simulink model "model_demo"  (R2023b)
settings: Solver=VariableStepAuto  StartTime=0.0  StopTime=10.0  RelTol=1e-3
undefined symbols (not defined in the file): DiscIntNeverNeededParam, magnitude, Newton, Raphson
libraries: simulink x61, slpidlib x19
(part 1 of 3)
settings Model: Creator=OSCAR4  LastModifiedBy=OSCAR4

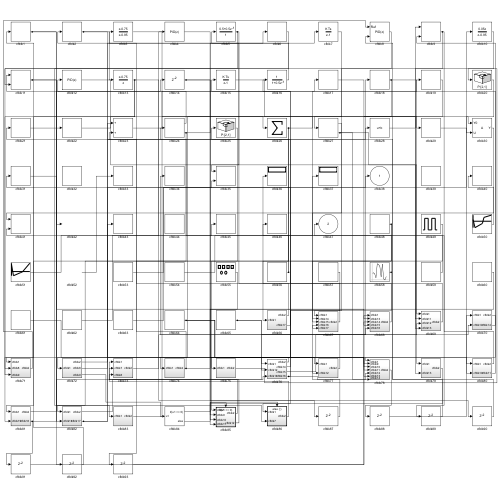
[thumbnail: Simulink's stored preview of the top-level diagram]
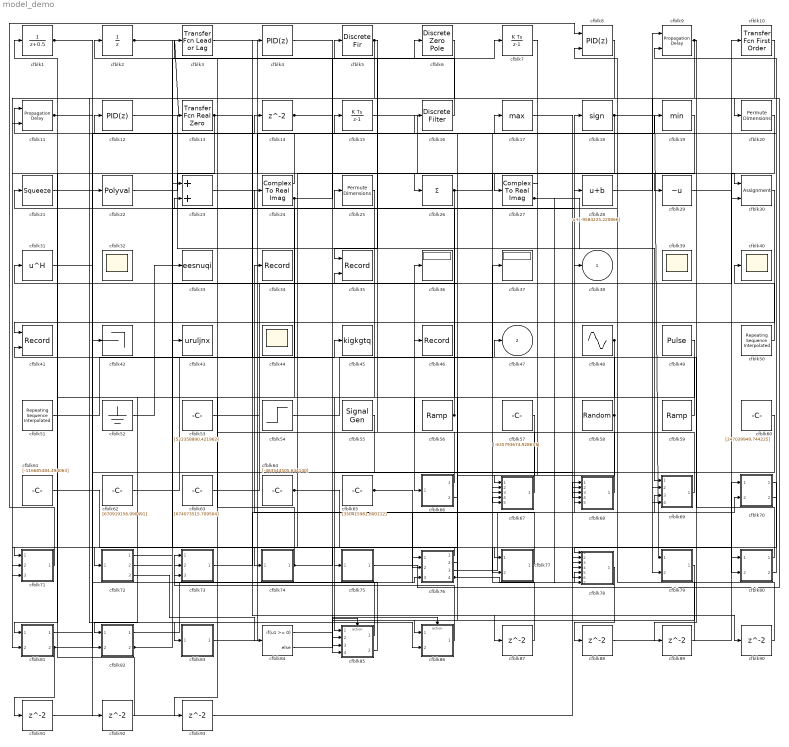
== system model_demo ==
  cfblk1 : DiscreteTransferFcn  SampleTime=1
  cfblk10 : simulink/Discrete/Transfer Fcn First Order  PoleZ=0.95  ICPrevOutput=0.0  DoSatur=off
  cfblk11 : PropagationDelay  SampleTime=1
  cfblk12 : slpidlib/PID Controller  Controller=PID  Form=Parallel  TimeDomain=Discrete-time  UseExternalTs=off  SampleTime=1  IntegratorMethod=Forward Euler  FilterMethod=Forward Euler  ControllerParametersSource=internal  P=1  I=1  UseKiTs=off  D=0  N=100  UseFilter=on  TunerSelectOption=Transfer Function Based (PID Tuner App)  InitialConditionSource=internal  InitialConditionForIntegrator=0  InitialConditionForFilter=0  DifferentiatorICPrevScaledInput=0  ExternalReset=none  TrackingMode=off  Kt=1  LimitOutput=off  SatLimitsSource=internal  UpperSaturationLimit=inf  LowerSaturationLimit=-inf  LinearizeAsGain=off  AntiWindupMode=none  Kb=1  LimitIntegrator=off  UpperIntegratorSaturationLimit=inf  LowerIntegratorSaturationLimit=-inf  POutMin=[]  POutMax=[]  IOutMin=[]  IOutMax=[]  DOutMin=[]  DOutMax=[]  NOutMin=[]  NOutMax=[]  SumOutMin=[]  SumOutMax=[]  SaturationOutMin=[]  SaturationOutMax=[]  PParamMin=[]  PParamMax=[]  IParamMin=[]  IParamMax=[]  DParamMin=[]  DParamMax=[]  NParamMin=[]  NParamMax=[]  KbParamMin=[]  KbParamMax=[]  KtParamMin=[]  KtParamMax=[]  KbOutMin=[]  KbOutMax=[]  KtOutMin=[]  KtOutMax=[]  IntegratorOutMin=[]  IntegratorOutMax=[]  FilterOutMin=[]  FilterOutMax=[]  SumI1OutMin=[]  SumI1OutMax=[]  SumI2OutMin=[]  SumI2OutMax=[]  SumI3OutMin=[]  SumI3OutMax=[]  SumI4OutMin=[]  SumI4OutMax=[]  SumDOutMin=[]  SumDOutMax=[]  DifferentiatorOutMin=[]  DifferentiatorOutMax=[]  FilterDiffOutCoefMin=[]  FilterDiffOutCoefMax=[]  ReciprocalOutMin=[]  ReciprocalOutMax=[]  SumDenOutMin=[]  SumDenOutMax=[]  SumNumOutMin=[]  SumNumOutMax=[]  DivideOutMin=[]  DivideOutMax=[]  UdiffTsProdOutMin=[]  UdiffTsProdOutMax=[]  NTsProdOutMin=[]  NTsProdOutMax=[]  UintegralTsProdOutMin=[]  UintegralTsProdOutMax=[]  UngainTsProdOutMin=[]  UngainTsProdOutMax=[]  ClampingZeroOutDataTypeStr=Inherit: Inherit via back propagation  ClampingZeroOutMin=[]  ClampingZeroOutMax=[]  FilterDenConstantOutDataTypeStr=Inherit: Inherit via back propagation  FilterDenConstantOutMin=[]  FilterDenConstantOutMax=[]  PCopyOutDataTypeStr=Inherit: Inherit via back propagation  PCopyOutMin=[]  PCopyOutMax=[]  NCopyOutDataTypeStr=Inherit: Inherit via back propagation  NCopyOutMin=[]  NCopyOutMax=[]  IntegratorContinuousStateAttributes=''  IntegratorStateMustResolveToSignalObject=off  IntegratorRTWStateStorageClass=Auto  FilterContinuousStateAttributes=''  FilterStateMustResolveToSignalObject=off  FilterRTWStateStorageClass=Auto  ParallelPVariant=InternalParameters  IdealPVariant=Disabled  IVariant=InternalParameters  DVariant=InternalParameters  IntegratorVariant=Discrete  SatVariant=Disabled  AWVariant=Passthrough  PCopyVariant=Disabled  TRVariant=Disabled  FdbkBlocksVariant=Forward  IdealPFdbkVariant=Disabled  SatFdbkVariant=Disabled  DerivativeFilterVariant=ForwardEulerFilter  NVariant=InternalParameters  NCopyVariant=Disabled  FilterICVariant=InternalICsFilter  IntegratorICVariant=InternalICs  ExternalResetVariant=Disabled  TRSumVariant=Passthrough  SumFdbkVariant=Disabled  SumVariant=Sum_PID  TsampFilterVariant=InternalTs  TsampNgainVariant=Passthrough  TsampIntegralVariant=Disabled_SignalSpec  ExternalSaturationOutDataTypeStr=Inherit: Same as second input
      settings: LibrarySourceBlock=simulink/Discrete/Discrete PID Controller
  cfblk13 : simulink/Discrete/Transfer Fcn Real Zero  ZeroZ=0.75  ICPrevInput=0.0  DoSatur=off
  cfblk{14,87..93} (8 alike) : Delay  SampleTime=1
  cfblk15 : DiscreteIntegrator  ICPrevOutput=DiscIntNeverNeededParam  ICPrevScaledInput=DiscIntNeverNeededParam
  cfblk16 : DiscreteFilter  SampleTime=1
  cfblk17 : MinMax  Function=max
  cfblk18 : Signum
  cfblk19 : MinMax
  cfblk2 : UnitDelay  HasFrameUpgradeWarning=on
  cfblk20 : PermuteDimensions
  cfblk21 : Squeeze
  cfblk22 : Polyval  Coefs=[ +2.081618890e-019, -1.441693666e-014, +4.719686976e-010, -8.536869453e-006, +1.621573104e-001, -8.087801117e+001 ]
  cfblk23 : Sum
  cfblk24 : ComplexToRealImag
  cfblk25 : PermuteDimensions
  cfblk26 : Sum  Inputs=+
  cfblk27 : ComplexToRealImag
  cfblk28 : Bias  Bias=[-9584225.220866]  SaturateOnIntegerOverflow=off
  cfblk29 : UnaryMinus
  cfblk3 : simulink/Discrete/Transfer Fcn Lead or Lag  PoleZ=0.95  ZeroZ=0.75  ICPrevOutput=0.0  ICPrevInput=0.0  DoSatur=off
  cfblk30 : Assignment  DiagnosticForDimensions=Warning  IndexOptions=Index vector (dialog)  Indices=1  OutputSizes=1
  cfblk31 : Math  Operator=hermitian
  cfblk{32,39..40,44} (4 alike) : Scope
      cfblk32 settings: Floating=on
      cfblk39 settings: Floating=on
      cfblk44 settings: Floating=on
  cfblk33 : ToWorkspace  VariableName=eesnuqi  SaveFormat=Timeseries  SampleTime=-1
  cfblk34 : Record  FileSettingsInternal="{\"entries\":[{\"content\":{\"excelSettings\":{\"content\":{},\"type\":\"Streamout.ExcelSettings\"}},\"type\":\"Streamout.FileSettingStorage\",\"uuid\":\"\"}],\"packageUris\":[\"http:\\/\\/schema.mathworks.com\\/mf0\\/streamout_blocks\\/R2020a\"],\"version\":\"1.0\"}"  SignalsInternal="{\"entries\":[{\"content\":{},\"type\":\"RecordBlkView.InputSignals\",\"uuid\":\"\"}],\"packageUris\":[\"http:\\/\\/schema.mathworks.com\\/mf0\\/streamout_blocks\\/R2020a\"],\"version\":\"1.0\"}"  VisualizationBindings="{\"sparklinesplugin\":{\"info\":[{\"bindingParametersList\":[],\"subplotID\":1}]}}"
  cfblk35 : Record  FileSettingsInternal="{\"entries\":[{\"content\":{\"excelSettings\":{\"content\":{},\"type\":\"Streamout.ExcelSettings\"}},\"type\":\"Streamout.FileSettingStorage\",\"uuid\":\"\"}],\"packageUris\":[\"http:\\/\\/schema.mathworks.com\\/mf0\\/streamout_blocks\\/R2020a\"],\"version\":\"1.0\"}"  Layout=[1 1]  SignalsInternal="{\"entries\":[{\"content\":{\"signals\":[{\"content\":{\"blockPath\":[],\"dimensions\":[1],\"domain\":\"\",\"lineColor\":\"#a2142f\",\"plots\":[1],\"port\":1,\"signalID\":7067,\"signalName\":\"XY Graph:1\"},\"type\":\"RecordBlkView.Signal\",\"uuid\":\"\"},{\"content\":{\"blockPath\":[],\"dimensions\":[1],\"domain\":\"\",\"lineColor\":\"#139fff\",\"plots\":[1],\"port\":2,\"signalID\":7070,\"signalName\":\"XY Graph:2\"},\"type\":\"RecordBlkView.Signal\",\"uuid\":\"\"}]},\"type\":\"RecordBlkView.InputSignals\",\"uuid\":\"\"}],\"packageUris\":[\"http:\\/\\/schema.mathworks.com\\/mf0\\/streamout_blocks\\/R2020a\"],\"version\":\"1.0\"}"  VisualizationBindings="{\"xyplotplugin\":{\"info\":[{\"series\":[{\"bindingParametersList\":[{\"parameter\":\"X-Axis\",\"signalID\":7067,\"signalName\":\"XY Graph:1\"},{\"parameter\":\"Y-Axis\",\"signalID\":7070,\"signalName\":\"XY Graph:2\"}],\"seriesID\":4920}],\"subplotID\":1}]}}"  CompatibilityTag=XY
  cfblk36 : Display
  cfblk37 : Display
  cfblk4 : slpidlib/PID Controller  Controller=PID  Form=Parallel  TimeDomain=Discrete-time  UseExternalTs=off  SampleTime=1  IntegratorMethod=Forward Euler  FilterMethod=Forward Euler  ControllerParametersSource=internal  P=1  I=1  UseKiTs=off  D=0  N=100  UseFilter=on  TunerSelectOption=Transfer Function Based (PID Tuner App)  InitialConditionSource=internal  InitialConditionForIntegrator=0  InitialConditionForFilter=0  DifferentiatorICPrevScaledInput=0  ExternalReset=none  TrackingMode=off  Kt=1  LimitOutput=off  SatLimitsSource=internal  UpperSaturationLimit=inf  LowerSaturationLimit=-inf  LinearizeAsGain=off  AntiWindupMode=none  Kb=1  LimitIntegrator=off  UpperIntegratorSaturationLimit=inf  LowerIntegratorSaturationLimit=-inf  POutMin=[]  POutMax=[]  IOutMin=[]  IOutMax=[]  DOutMin=[]  DOutMax=[]  NOutMin=[]  NOutMax=[]  SumOutMin=[]  SumOutMax=[]  SaturationOutMin=[]  SaturationOutMax=[]  PParamMin=[]  PParamMax=[]  IParamMin=[]  IParamMax=[]  DParamMin=[]  DParamMax=[]  NParamMin=[]  NParamMax=[]  KbParamMin=[]  KbParamMax=[]  KtParamMin=[]  KtParamMax=[]  KbOutMin=[]  KbOutMax=[]  KtOutMin=[]  KtOutMax=[]  IntegratorOutMin=[]  IntegratorOutMax=[]  FilterOutMin=[]  FilterOutMax=[]  SumI1OutMin=[]  SumI1OutMax=[]  SumI2OutMin=[]  SumI2OutMax=[]  SumI3OutMin=[]  SumI3OutMax=[]  SumI4OutMin=[]  SumI4OutMax=[]  SumDOutMin=[]  SumDOutMax=[]  DifferentiatorOutMin=[]  DifferentiatorOutMax=[]  FilterDiffOutCoefMin=[]  FilterDiffOutCoefMax=[]  ReciprocalOutMin=[]  ReciprocalOutMax=[]  SumDenOutMin=[]  SumDenOutMax=[]  SumNumOutMin=[]  SumNumOutMax=[]  DivideOutMin=[]  DivideOutMax=[]  UdiffTsProdOutMin=[]  UdiffTsProdOutMax=[]  NTsProdOutMin=[]  NTsProdOutMax=[]  UintegralTsProdOutMin=[]  UintegralTsProdOutMax=[]  UngainTsProdOutMin=[]  UngainTsProdOutMax=[]  ClampingZeroOutDataTypeStr=Inherit: Inherit via back propagation  ClampingZeroOutMin=[]  ClampingZeroOutMax=[]  FilterDenConstantOutDataTypeStr=Inherit: Inherit via back propagation  FilterDenConstantOutMin=[]  FilterDenConstantOutMax=[]  PCopyOutDataTypeStr=Inherit: Inherit via back propagation  PCopyOutMin=[]  PCopyOutMax=[]  NCopyOutDataTypeStr=Inherit: Inherit via back propagation  NCopyOutMin=[]  NCopyOutMax=[]  IntegratorContinuousStateAttributes=''  IntegratorStateMustResolveToSignalObject=off  IntegratorRTWStateStorageClass=Auto  FilterContinuousStateAttributes=''  FilterStateMustResolveToSignalObject=off  FilterRTWStateStorageClass=Auto  ParallelPVariant=InternalParameters  IdealPVariant=Disabled  IVariant=InternalParameters  DVariant=InternalParameters  IntegratorVariant=Discrete  SatVariant=Disabled  AWVariant=Passthrough  PCopyVariant=Disabled  TRVariant=Disabled  FdbkBlocksVariant=Forward  IdealPFdbkVariant=Disabled  SatFdbkVariant=Disabled  DerivativeFilterVariant=ForwardEulerFilter  NVariant=InternalParameters  NCopyVariant=Disabled  FilterICVariant=InternalICsFilter  IntegratorICVariant=InternalICs  ExternalResetVariant=Disabled  TRSumVariant=Passthrough  SumFdbkVariant=Disabled  SumVariant=Sum_PID  TsampFilterVariant=InternalTs  TsampNgainVariant=Passthrough  TsampIntegralVariant=Disabled_SignalSpec  ExternalSaturationOutDataTypeStr=Inherit: Same as second input
      settings: LibrarySourceBlock=simulink/Discrete/Discrete PID Controller
  cfblk41 : Record  FileSettingsInternal="{\"entries\":[{\"content\":{\"excelSettings\":{\"content\":{},\"type\":\"Streamout.ExcelSettings\"}},\"type\":\"Streamout.FileSettingStorage\",\"uuid\":\"\"}],\"packageUris\":[\"http:\\/\\/schema.mathworks.com\\/mf0\\/streamout_blocks\\/R2020a\"],\"version\":\"1.0\"}"  Layout=[1 1]  SignalsInternal="{\"entries\":[{\"content\":{\"signals\":[{\"content\":{\"blockPath\":[],\"dimensions\":[1],\"domain\":\"\",\"lineColor\":\"#a2142f\",\"plots\":[1],\"port\":1,\"signalID\":7075,\"signalName\":\"XY Graph:1\"},\"type\":\"RecordBlkView.Signal\",\"uuid\":\"\"},{\"content\":{\"blockPath\":[],\"dimensions\":[1],\"domain\":\"\",\"lineColor\":\"#139fff\",\"plots\":[1],\"port\":2,\"signalID\":7078,\"signalName\":\"XY Graph:2\"},\"type\":\"RecordBlkView.Signal\",\"uuid\":\"\"}]},\"type\":\"RecordBlkView.InputSignals\",\"uuid\":\"\"}],\"packageUris\":[\"http:\\/\\/schema.mathworks.com\\/mf0\\/streamout_blocks\\/R2020a\"],\"version\":\"1.0\"}"  VisualizationBindings="{\"xyplotplugin\":{\"info\":[{\"series\":[{\"bindingParametersList\":[{\"parameter\":\"X-Axis\",\"signalID\":7075,\"signalName\":\"XY Graph:1\"},{\"parameter\":\"Y-Axis\",\"signalID\":7078,\"signalName\":\"XY Graph:2\"}],\"seriesID\":57556}],\"subplotID\":1}]}}"  CompatibilityTag=XY
  cfblk42 : Terminator
  cfblk43 : ToWorkspace  VariableName=uruljnx  SaveFormat=Timeseries  SampleTime=-1
  cfblk45 : ToWorkspace  VariableName=kigkgtq  SaveFormat=Timeseries  SampleTime=-1
  cfblk46 : Record  FileSettingsInternal="{\"entries\":[{\"content\":{\"excelSettings\":{\"content\":{},\"type\":\"Streamout.ExcelSettings\"}},\"type\":\"Streamout.FileSettingStorage\",\"uuid\":\"\"}],\"packageUris\":[\"http:\\/\\/schema.mathworks.com\\/mf0\\/streamout_blocks\\/R2020a\"],\"version\":\"1.0\"}"  SignalsInternal="{\"entries\":[{\"content\":{},\"type\":\"RecordBlkView.InputSignals\",\"uuid\":\"\"}],\"packageUris\":[\"http:\\/\\/schema.mathworks.com\\/mf0\\/streamout_blocks\\/R2020a\"],\"version\":\"1.0\"}"  VisualizationBindings="{\"sparklinesplugin\":{\"info\":[{\"bindingParametersList\":[],\"subplotID\":1}]}}"
  cfblk48 : Sin  Amplitude=[-114509519.258269]  Bias=[-794873402.533103]  SampleTime=0
  cfblk49 : DiscretePulseGenerator  PulseType=Time based  Amplitude=[983212804.786086]  Period=[36735637.140367]  PulseWidth=5  PhaseDelay=[7.000000]
  cfblk5 : DiscreteFir  SampleTime=1
  cfblk50 : simulink/Sources/Repeating Sequence Interpolated  OutValues=[202675780.097570, -805155043.980317, -271725127.779501, 482624865.151505, 771303494.204872]  TimeValues=[0 0.1 0.5 0.6 1].'  LookUpMeth=Interpolation-Use End Values  tsamp=0.01  OutMin=[]  OutMax=[]  OutDataTypeStr=double  OutputDataTypeScalingMode=double  OutDataType=fixdt(0,8)  OutScaling=2^-10
  cfblk51 : simulink/Sources/Repeating Sequence Interpolated  OutValues=[789067957.080977, -455495792.936879, -89334232.326252, -42277899.737208, 973363783.120108]  TimeValues=[0 0.1 0.5 0.6 1].'  LookUpMeth=Use Input Nearest  tsamp=0.01  OutMin=[]  OutMax=[]  OutDataTypeStr=double  OutputDataTypeScalingMode=double  OutDataType=fixdt(0,8)  OutScaling=2^-10
  cfblk52 : Ground
  cfblk53 : Constant  Value=[522358890.421962]  SampleTime=1
  cfblk54 : Step  Time=[46.000000]  Before=[-523718207.875303]  After=[-24350030.205386]  SampleTime=0
  cfblk55 : SignalGenerator  WaveForm=square  Amplitude=[-796796388.431392]
  cfblk56 : simulink/Sources/Ramp  slope=[-5461.696491]  start=[15.070192]  InitialOutput=[-543328.774158]
  cfblk57 : Constant  Value=[-635793674.928637]  SampleTime=1
  cfblk58 : RandomNumber  Mean=[33488.965661]  Variance=[98341.878984]  Seed=[473972234.000000]  SampleTime=0.1
  cfblk59 : simulink/Sources/Ramp  slope=[-1343.464601]  start=[25.451942]  InitialOutput=[649478.584814]
  cfblk6 : DiscreteZeroPole  Poles=[0 0.5]  Gain=1
  cfblk60 : Constant  Value=[247039949.744225]  SampleTime=1
  cfblk61 : Constant  Value=[-116685484.494063]  SampleTime=1
  cfblk62 : Constant  Value=[670919156.990491]  SampleTime=1
  cfblk63 : Constant  Value=[674073515.709504]  SampleTime=1
  cfblk64 : Constant  Value=[-463544505.644140]  SampleTime=1
  cfblk65 : Constant  Value=[350415981.600112]  SampleTime=1
  cfblk66 : Subsystem
  cfblk67 : Subsystem
  cfblk68 : Subsystem
  cfblk69 : Subsystem
  cfblk7 : DiscreteIntegrator  ICPrevOutput=DiscIntNeverNeededParam  ICPrevScaledInput=DiscIntNeverNeededParam
  cfblk70 : Subsystem
  cfblk71 : Subsystem
  cfblk72 : Subsystem
  cfblk73 : Subsystem
  cfblk74 : Subsystem
  cfblk75 : Subsystem
  cfblk76 : Subsystem
  cfblk77 : Subsystem
  cfblk78 : Subsystem
  cfblk79 : Subsystem
  cfblk8 : slpidlib/PID Controller (2DOF)  Controller=PID  Form=Parallel  TimeDomain=Discrete-time  UseExternalTs=off  SampleTime=1  IntegratorMethod=Forward Euler  FilterMethod=Forward Euler  ControllerParametersSource=internal  P=1  I=1  UseKiTs=off  D=0  N=100  UseFilter=on  b=1  c=1  TunerSelectOption=Transfer Function Based (PID Tuner App)  InitialConditionSource=internal  InitialConditionForIntegrator=0  InitialConditionForFilter=0  DifferentiatorICPrevScaledInput=0  ExternalReset=none  TrackingMode=off  Kt=1  LimitOutput=off  SatLimitsSource=internal  UpperSaturationLimit=inf  LowerSaturationLimit=-inf  LinearizeAsGain=off  AntiWindupMode=none  Kb=1  LimitIntegrator=off  UpperIntegratorSaturationLimit=inf  LowerIntegratorSaturationLimit=-inf  POutMin=[]  POutMax=[]  IOutMin=[]  IOutMax=[]  DOutMin=[]  DOutMax=[]  NOutMin=[]  NOutMax=[]  bOutMin=[]  bOutMax=[]  cOutMin=[]  cOutMax=[]  SumOutMin=[]  SumOutMax=[]  SaturationOutMin=[]  SaturationOutMax=[]  PParamMin=[]  PParamMax=[]  IParamMin=[]  IParamMax=[]  DParamMin=[]  DParamMax=[]  NParamMin=[]  NParamMax=[]  bParamMin=[]  bParamMax=[]  cParamMin=[]  cParamMax=[]  KbParamMin=[]  KbParamMax=[]  KtParamMin=[]  KtParamMax=[]  KbOutMin=[]  KbOutMax=[]  KtOutMin=[]  KtOutMax=[]  IntegratorOutMin=[]  IntegratorOutMax=[]  FilterOutMin=[]  FilterOutMax=[]  SumI1OutMin=[]  SumI1OutMax=[]  SumI2OutMin=[]  SumI2OutMax=[]  SumI3OutMin=[]  SumI3OutMax=[]  SumI4OutMin=[]  SumI4OutMax=[]  SumDOutMin=[]  SumDOutMax=[]  Sum1OutMin=[]  Sum1OutMax=[]  Sum2OutMin=[]  Sum2OutMax=[]  Sum3OutMin=[]  Sum3OutMax=[]  DifferentiatorOutMin=[]  DifferentiatorOutMax=[]  FilterDiffOutCoefMin=[]  FilterDiffOutCoefMax=[]  ReciprocalOutMin=[]  ReciprocalOutMax=[]  SumDenOutMin=[]  SumDenOutMax=[]  SumNumOutMin=[]  SumNumOutMax=[]  DivideOutMin=[]  DivideOutMax=[]  UdiffTsProdOutMin=[]  UdiffTsProdOutMax=[]  NTsProdOutMin=[]  NTsProdOutMax=[]  UintegralTsProdOutMin=[]  UintegralTsProdOutMax=[]  UngainTsProdOutMin=[]  UngainTsProdOutMax=[]  ClampingZeroOutDataTypeStr=Inherit: Inherit via back propagation  ClampingZeroOutMin=[]  ClampingZeroOutMax=[]  FilterDenConstantOutDataTypeStr=Inherit: Inherit via back propagation  FilterDenConstantOutMin=[]  FilterDenConstantOutMax=[]  PCopyOutDataTypeStr=Inherit: Inherit via back propagation  PCopyOutMin=[]  PCopyOutMax=[]  NCopyOutDataTypeStr=Inherit: Inherit via back propagation  NCopyOutMin=[]  NCopyOutMax=[]  IntegratorContinuousStateAttributes=''  IntegratorStateMustResolveToSignalObject=off  IntegratorRTWStateStorageClass=Auto  FilterContinuousStateAttributes=''  FilterStateMustResolveToSignalObject=off  FilterRTWStateStorageClass=Auto  ParallelPVariant=InternalParameters  IdealPVariant=Disabled  IVariant=InternalParameters  DVariant=InternalParameters  bVariant=InternalParameters  cVariant=InternalParameters  IntegratorVariant=Discrete  SatVariant=Disabled  AWVariant=Passthrough  PCopyVariant=Disabled  TRVariant=Disabled  FdbkBlocksVariant=Forward  IdealPFdbkVariant=Disabled  SatFdbkVariant=Disabled  DerivativeFilterVariant=ForwardEulerFilter  NVariant=InternalParameters  NCopyVariant=Disabled  FilterICVariant=InternalICsFilter  IntegratorICVariant=InternalICs  ExternalResetVariant=Disabled  TRSumVariant=Passthrough  SumFdbkVariant=Disabled  SumVariant=Sum_PID  TsampFilterVariant=InternalTs  TsampNgainVariant=Passthrough  TsampIntegralVariant=Disabled_SignalSpec  ExternalSaturationOutDataTypeStr=Inherit: Same as second input
      settings: LibrarySourceBlock=simulink/Discrete/Discrete PID Controller (2DOF)
  cfblk80 : Subsystem
  cfblk81 : Subsystem
  cfblk82 : Subsystem
  cfblk83 : Subsystem
  cfblk84 : If  IfExpression=u1 >= 0  SampleTime=1
  cfblk85 : Subsystem  TreatAsAtomicUnit=on
  cfblk86 : Subsystem  TreatAsAtomicUnit=on
  cfblk9 : PropagationDelay  SampleTime=1
  cfblk38 : Outport
  cfblk47 : Outport  Port=2
  wires:
  cfblk63/1 -> cfblk18/1
  cfblk85/1(cfblk2) -> cfblk73/1(cfblk1)
  cfblk80/1(cfblk2) -> cfblk47/1
  cfblk76/1(cfblk2) -> cfblk72/1(cfblk1)
  cfblk25/1 -> cfblk85/1(cfblk1)
  cfblk54/1 -> cfblk37/1
  cfblk23/1 -> cfblk26/1
  cfblk18/1 -> cfblk79/1(cfblk1), cfblk68/4(cfblk15)
  cfblk83/1(cfblk2) -> cfblk17/1
  cfblk7/1 -> cfblk27/1
  cfblk6/1 -> cfblk83/1(cfblk1)
  cfblk52/1 -> cfblk33/1
  cfblk27/1 -> cfblk41/1
  cfblk12/1 -> cfblk69/1(cfblk1)
  cfblk80/2(cfblk11) -> cfblk15/1
  cfblk69/1(cfblk2) -> cfblk36/1
  cfblk2/1 -> cfblk13/1, cfblk77/2(cfblk12)
  cfblk77/1(cfblk2) -> cfblk34/1
  cfblk59/1 -> cfblk24/1
  cfblk22/1 -> cfblk30/1
  cfblk72/1(cfblk2) -> cfblk43/1
  cfblk72/2(cfblk8) -> cfblk28/1
  cfblk20/1 -> cfblk30/2
  cfblk71/1(cfblk2) -> cfblk8/1
  cfblk48/1 -> cfblk66/1(cfblk1), cfblk67/5(cfblk17)
  cfblk9/1 -> cfblk69/4(cfblk13), cfblk89/1
  cfblk5/1 -> cfblk35/1, cfblk81/2(cfblk15)
  cfblk53/1 -> cfblk10/1
  cfblk72/3(cfblk9) -> cfblk84/1
  cfblk75/1(cfblk2) -> cfblk20/1
  cfblk24/1 -> cfblk12/1
  cfblk15/1 -> cfblk79/2(cfblk13)
  cfblk50/1 -> cfblk40/1
  cfblk19/1 -> cfblk74/1(cfblk1)
  cfblk85/2(cfblk12) -> cfblk73/2(cfblk7)
  cfblk74/1(cfblk2) -> cfblk3/1, cfblk77/1(cfblk1)
  cfblk17/1 -> cfblk29/1
  cfblk11/1 -> cfblk42/1, cfblk86/2(cfblk7)
  cfblk56/1 -> cfblk5/1, cfblk46/1
  cfblk58/1 -> cfblk41/2, cfblk71/2(cfblk8)
  cfblk70/1(cfblk2) -> cfblk78/1(cfblk1)
  cfblk10/1 -> cfblk67/1(cfblk1)
  cfblk29/1 -> cfblk80/1(cfblk1)
  cfblk1/1 -> cfblk22/1, cfblk68/2(cfblk13)
  cfblk3/1 -> cfblk67/2(cfblk14)
  cfblk67/1(cfblk2) -> cfblk16/1
  cfblk79/1(cfblk2) -> cfblk85/2(cfblk9)
  cfblk28/1 -> cfblk9/1
  cfblk73/1(cfblk2) -> cfblk70/2(cfblk13)
  cfblk16/1 -> cfblk2/1
  cfblk30/1 -> cfblk67/3(cfblk15)
  cfblk14/1 -> cfblk78/4(cfblk11), cfblk90/1
  cfblk76/2(cfblk14) -> cfblk11/1
  cfblk8/1 -> cfblk11/2
  cfblk24/2 -> cfblk82/1(cfblk1), cfblk6/1
  cfblk65/1 -> cfblk76/1(cfblk1), cfblk68/5(cfblk16)
  cfblk13/1 -> cfblk71/1(cfblk1), cfblk71/3(cfblk9), cfblk87/1
  cfblk49/1 -> cfblk86/1(cfblk1)
  cfblk62/1 -> cfblk4/1
  cfblk51/1 -> cfblk45/1
  cfblk31/1 -> cfblk82/2(cfblk16)
  cfblk61/1 -> cfblk75/1(cfblk1)
  cfblk27/2 -> cfblk69/2(cfblk11), cfblk78/7(cfblk14)
  cfblk60/1 -> cfblk85/3(cfblk10)
  cfblk68/1(cfblk2) -> cfblk23/2
  cfblk26/1 -> cfblk19/1, cfblk81/1(cfblk1), cfblk93/1
  cfblk66/1(cfblk2) -> cfblk25/1
  cfblk82/1(cfblk2) -> cfblk69/3(cfblk12)
  cfblk76/3(cfblk15) -> cfblk38/1
  cfblk82/2(cfblk17) -> cfblk7/1, cfblk35/2
  cfblk76/4(cfblk16) -> cfblk21/1, cfblk78/5(cfblk12)
  cfblk4/1 -> cfblk78/2(cfblk9)
  cfblk55/1 -> cfblk85/4(cfblk11)
  cfblk81/1(cfblk2) -> cfblk14/1
  cfblk70/2(cfblk14) -> cfblk9/2
  cfblk86/1(cfblk2) -> cfblk73/3(cfblk8)
  cfblk81/2(cfblk16) -> cfblk76/3(cfblk13), cfblk91/1
  cfblk57/1 -> cfblk76/2(cfblk12)
  cfblk64/1 -> cfblk78/3(cfblk10), cfblk80/2(cfblk10), cfblk78/6(cfblk13)
  cfblk66/2(cfblk17) -> cfblk31/1
  cfblk84/1 -> cfblk85/Action
  cfblk84/2 -> cfblk86/Action
  cfblk87/1 -> cfblk67/4(cfblk16)
  cfblk78/1(cfblk2) -> cfblk88/1
  cfblk88/1 -> cfblk70/1(cfblk1)
  cfblk89/1 -> cfblk8/2
  cfblk90/1 -> cfblk23/1
  cfblk91/1 -> cfblk68/1(cfblk1)
  cfblk21/1 -> cfblk92/1
  cfblk92/1 -> cfblk1/1
  cfblk93/1 -> cfblk68/3(cfblk14)

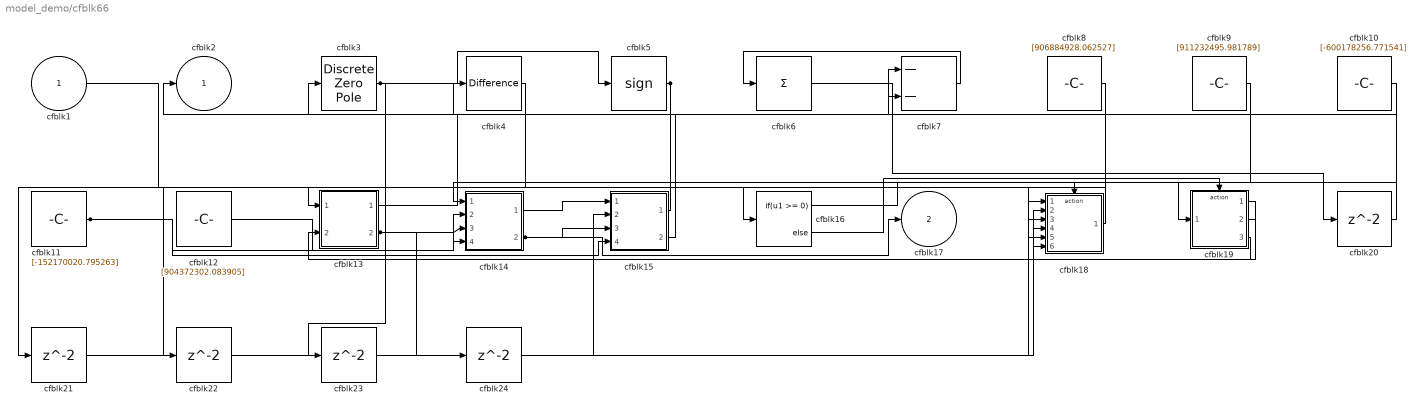
== system model_demo/cfblk66 ==
  cfblk1 : Inport
  cfblk10 : Constant  Value=[-600178256.771541]  SampleTime=1
  cfblk11 : Constant  Value=[-152170020.795263]  SampleTime=1
  cfblk12 : Constant  Value=[904372302.083905]  SampleTime=1
  cfblk13 : Subsystem
  cfblk14 : Subsystem
  cfblk15 : Subsystem
  cfblk16 : If  IfExpression=u1 >= 0  SampleTime=1
  cfblk18 : Subsystem  TreatAsAtomicUnit=on
  cfblk19 : Subsystem  TreatAsAtomicUnit=on
  cfblk{20..24} (5 alike) : Delay  SampleTime=1
  cfblk3 : DiscreteZeroPole  Poles=[0 0.5]  Gain=1
  cfblk4 : simulink/Discrete/Difference  ICPrevInput=0.0  OutMin=[]  OutMax=[]  OutDataTypeStr=Inherit: Inherit via back propagation  OutDataType=fixdt(1, 16)  OutScaling=2^-10  DoSatur=off
  cfblk5 : Signum
  cfblk6 : Sum  Inputs=+
  cfblk7 : Sum  Inputs=--
  cfblk8 : Constant  Value=[906884928.062527]  SampleTime=1
  cfblk9 : Constant  Value=[911232495.981789]  SampleTime=1
  cfblk2 : Outport
  cfblk17 : Outport  Port=2
  wires:
  cfblk15/1(cfblk2) -> cfblk2/1
  cfblk5/1 -> cfblk21/1, cfblk22/1
  cfblk3/1 -> cfblk5/1, cfblk23/1
  cfblk4/1 -> cfblk13/1(cfblk1)
  cfblk13/1(cfblk2) -> cfblk7/1
  cfblk9/1 -> cfblk14/1(cfblk1)
  cfblk8/1 -> cfblk16/1
  cfblk11/1 -> cfblk14/2(cfblk6), cfblk15/4(cfblk15)
  cfblk13/2(cfblk7) -> cfblk14/3(cfblk7), cfblk24/1
  cfblk7/1 -> cfblk6/1
  cfblk15/2(cfblk16) -> cfblk3/1
  cfblk14/1(cfblk2) -> cfblk15/1(cfblk1)
  cfblk12/1 -> cfblk14/4(cfblk8)
  cfblk14/2(cfblk9) -> cfblk17/1, cfblk15/3(cfblk14)
  cfblk18/1(cfblk2) -> cfblk4/1
  cfblk19/1(cfblk2) -> cfblk18/2(cfblk6)
  cfblk10/1 -> cfblk19/1(cfblk1)
  cfblk1/1 -> cfblk18/3(cfblk7)
  cfblk19/2(cfblk6) -> cfblk18/4(cfblk8)
  cfblk19/3(cfblk7) -> cfblk13/2(cfblk6)
  cfblk16/1 -> cfblk18/Action
  cfblk16/2 -> cfblk19/Action
  cfblk6/1 -> cfblk20/1
  cfblk20/1 -> cfblk7/2
  cfblk21/1 -> cfblk18/1(cfblk1)
  cfblk22/1 -> cfblk18/5(cfblk9)
  cfblk23/1 -> cfblk15/2(cfblk13)
  cfblk24/1 -> cfblk18/6(cfblk10)

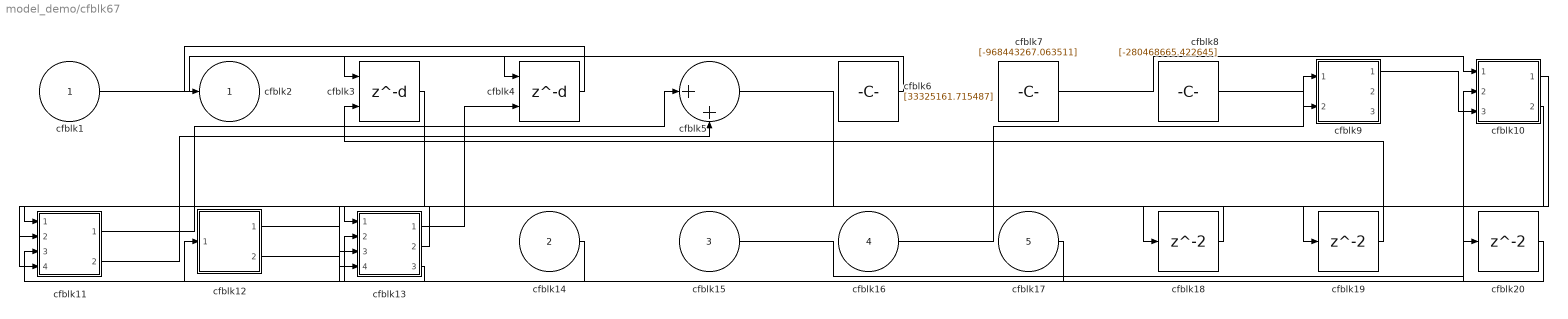
== system model_demo/cfblk67 ==
  cfblk1 : Inport
  cfblk14 : Inport  Port=2
  cfblk15 : Inport  Port=3
  cfblk16 : Inport  Port=4
  cfblk17 : Inport  Port=5
  cfblk10 : Subsystem
  cfblk11 : Subsystem
  cfblk12 : Subsystem
  cfblk13 : Subsystem
  cfblk18 : Delay  SampleTime=1
  cfblk19 : Delay  SampleTime=1
  cfblk20 : Delay  SampleTime=1
  cfblk3 : Delay  DelayLengthSource=Input port  SampleTime=1
      settings: InputPortMap=u0,p1
  cfblk4 : Delay  DelayLengthSource=Input port  SampleTime=1
      settings: InputPortMap=u0,p1
  cfblk5 : Sum  Inputs=|++
  cfblk6 : Constant  Value=[33325161.715487]  SampleTime=1
  cfblk7 : Constant  Value=[-968443267.063511]  SampleTime=1
  cfblk8 : Constant  Value=[-280468665.422645]  SampleTime=1
  cfblk9 : Subsystem
  cfblk2 : Outport
  wires:
  cfblk1/1 -> cfblk4/1
  cfblk3/1 -> cfblk13/1(cfblk1)
  cfblk4/1 -> cfblk2/1
  cfblk16/1 -> cfblk9/1(cfblk1)
  cfblk6/1 -> cfblk3/1
  cfblk14/1 -> cfblk13/2(cfblk13)
  cfblk8/1 -> cfblk9/2(cfblk5)
  cfblk13/1(cfblk2) -> cfblk4/2
  cfblk7/1 -> cfblk10/1(cfblk1)
  cfblk13/2(cfblk16) -> cfblk11/1(cfblk1)
  cfblk13/3(cfblk17) -> cfblk12/1(cfblk1)
  cfblk15/1 -> cfblk10/2(cfblk8)
  cfblk9/1(cfblk2) -> cfblk10/3(cfblk9)
  cfblk17/1 -> cfblk11/3(cfblk14)
  cfblk11/1(cfblk2) -> cfblk5/1
  cfblk10/1(cfblk2) -> cfblk13/4(cfblk15)
  cfblk10/2(cfblk10) -> cfblk11/4(cfblk15)
  cfblk11/2(cfblk16) -> cfblk5/2
  cfblk5/1 -> cfblk18/1
  cfblk18/1 -> cfblk11/2(cfblk13)
  cfblk12/1(cfblk2) -> cfblk19/1
  cfblk19/1 -> cfblk3/2
  cfblk12/2(cfblk7) -> cfblk20/1
  cfblk20/1 -> cfblk13/3(cfblk14)

== system model_demo/cfblk68 ==
  cfblk1 : Inport
  cfblk13 : Inport  Port=2
  cfblk14 : Inport  Port=3
  cfblk15 : Inport  Port=4
  cfblk16 : Inport  Port=5
  cfblk10 : Subsystem
  cfblk11 : Subsystem
  cfblk12 : Subsystem
  cfblk3 : slpidlib/PID Controller  Controller=PID  Form=Parallel  TimeDomain=Discrete-time  UseExternalTs=off  SampleTime=1  IntegratorMethod=Forward Euler  FilterMethod=Forward Euler  ControllerParametersSource=internal  P=1  I=1  UseKiTs=off  D=0  N=100  UseFilter=on  TunerSelectOption=Transfer Function Based (PID Tuner App)  InitialConditionSource=internal  InitialConditionForIntegrator=0  InitialConditionForFilter=0  DifferentiatorICPrevScaledInput=0  ExternalReset=none  TrackingMode=off  Kt=1  LimitOutput=off  SatLimitsSource=internal  UpperSaturationLimit=inf  LowerSaturationLimit=-inf  LinearizeAsGain=off  AntiWindupMode=none  Kb=1  LimitIntegrator=off  UpperIntegratorSaturationLimit=inf  LowerIntegratorSaturationLimit=-inf  POutMin=[]  POutMax=[]  IOutMin=[]  IOutMax=[]  DOutMin=[]  DOutMax=[]  NOutMin=[]  NOutMax=[]  SumOutMin=[]  SumOutMax=[]  SaturationOutMin=[]  SaturationOutMax=[]  PParamMin=[]  PParamMax=[]  IParamMin=[]  IParamMax=[]  DParamMin=[]  DParamMax=[]  NParamMin=[]  NParamMax=[]  KbParamMin=[]  KbParamMax=[]  KtParamMin=[]  KtParamMax=[]  KbOutMin=[]  KbOutMax=[]  KtOutMin=[]  KtOutMax=[]  IntegratorOutMin=[]  IntegratorOutMax=[]  FilterOutMin=[]  FilterOutMax=[]  SumI1OutMin=[]  SumI1OutMax=[]  SumI2OutMin=[]  SumI2OutMax=[]  SumI3OutMin=[]  SumI3OutMax=[]  SumI4OutMin=[]  SumI4OutMax=[]  SumDOutMin=[]  SumDOutMax=[]  DifferentiatorOutMin=[]  DifferentiatorOutMax=[]  FilterDiffOutCoefMin=[]  FilterDiffOutCoefMax=[]  ReciprocalOutMin=[]  ReciprocalOutMax=[]  SumDenOutMin=[]  SumDenOutMax=[]  SumNumOutMin=[]  SumNumOutMax=[]  DivideOutMin=[]  DivideOutMax=[]  UdiffTsProdOutMin=[]  UdiffTsProdOutMax=[]  NTsProdOutMin=[]  NTsProdOutMax=[]  UintegralTsProdOutMin=[]  UintegralTsProdOutMax=[]  UngainTsProdOutMin=[]  UngainTsProdOutMax=[]  ClampingZeroOutDataTypeStr=Inherit: Inherit via back propagation  ClampingZeroOutMin=[]  ClampingZeroOutMax=[]  FilterDenConstantOutDataTypeStr=Inherit: Inherit via back propagation  FilterDenConstantOutMin=[]  FilterDenConstantOutMax=[]  PCopyOutDataTypeStr=Inherit: Inherit via back propagation  PCopyOutMin=[]  PCopyOutMax=[]  NCopyOutDataTypeStr=Inherit: Inherit via back propagation  NCopyOutMin=[]  NCopyOutMax=[]  IntegratorContinuousStateAttributes=''  IntegratorStateMustResolveToSignalObject=off  IntegratorRTWStateStorageClass=Auto  FilterContinuousStateAttributes=''  FilterStateMustResolveToSignalObject=off  FilterRTWStateStorageClass=Auto  ParallelPVariant=InternalParameters  IdealPVariant=Disabled  IVariant=InternalParameters  DVariant=InternalParameters  IntegratorVariant=Discrete  SatVariant=Disabled  AWVariant=Passthrough  PCopyVariant=Disabled  TRVariant=Disabled  FdbkBlocksVariant=Forward  IdealPFdbkVariant=Disabled  SatFdbkVariant=Disabled  DerivativeFilterVariant=ForwardEulerFilter  NVariant=InternalParameters  NCopyVariant=Disabled  FilterICVariant=InternalICsFilter  IntegratorICVariant=InternalICs  ExternalResetVariant=Disabled  TRSumVariant=Passthrough  SumFdbkVariant=Disabled  SumVariant=Sum_PID  TsampFilterVariant=InternalTs  TsampNgainVariant=Passthrough  TsampIntegralVariant=Disabled_SignalSpec  ExternalSaturationOutDataTypeStr=Inherit: Same as second input
      settings: LibrarySourceBlock=simulink/Discrete/Discrete PID Controller
  cfblk4 : DiscreteIntegrator  ICPrevOutput=DiscIntNeverNeededParam  ICPrevScaledInput=DiscIntNeverNeededParam
  cfblk5 : DiscreteZeroPole  Poles=[0 0.5]  Gain=1
  cfblk6 : Trigonometry
  cfblk7 : ComplexToRealImag
  cfblk8 : UnaryMinus
  cfblk9 : Constant  Value=[-547815006.081445]  SampleTime=1
  cfblk2 : Outport
  wires:
  cfblk8/1 -> cfblk11/1(cfblk1)
  cfblk14/1 -> cfblk3/1
  cfblk16/1 -> cfblk4/1
  cfblk10/1(cfblk2) -> cfblk8/1
  cfblk5/1 -> cfblk10/1(cfblk1)
  cfblk15/1 -> cfblk5/1
  cfblk1/1 -> cfblk10/2(cfblk8)
  cfblk9/1 -> cfblk7/1
  cfblk4/1 -> cfblk6/1
  cfblk11/1(cfblk2) -> cfblk12/1(cfblk1)
  cfblk10/2(cfblk9) -> cfblk2/1
  cfblk10/3(cfblk10) -> cfblk12/2(cfblk8)
  cfblk3/1 -> cfblk12/3(cfblk9)

== system model_demo/cfblk69 ==
  cfblk1 : Inport
  cfblk11 : Inport  Port=2
  cfblk12 : Inport  Port=3
  cfblk13 : Inport  Port=4
  cfblk10 : Subsystem
  cfblk14 : Delay  SampleTime=1
  cfblk3 : Delay  ShowEnablePort=on  SampleTime=1
      settings: InputPortMap=u0,e6
  cfblk4 : Trigonometry
  cfblk5 : Constant  Value=[283766932.316221]  SampleTime=1
  cfblk6 : Constant  Value=[391082384.786132]  SampleTime=1
  cfblk7 : Constant  Value=[-806418958.515881]  SampleTime=1
  cfblk8 : Subsystem
  cfblk9 : Subsystem
  cfblk2 : Outport
  wires:
  cfblk4/1 -> cfblk10/1(cfblk1)
  cfblk6/1 -> cfblk8/1(cfblk1)
  cfblk12/1 -> cfblk4/1
  cfblk10/1(cfblk2) -> cfblk9/1(cfblk1)
  cfblk11/1 -> cfblk3/2
  cfblk3/1 -> cfblk10/2(cfblk8)
  cfblk5/1 -> cfblk9/2(cfblk12)
  cfblk13/1 -> cfblk8/2(cfblk8)
  cfblk10/2(cfblk9) -> cfblk2/1
  cfblk7/1 -> cfblk8/3(cfblk9)
  cfblk9/2(cfblk13) -> cfblk8/4(cfblk10)
  cfblk1/1 -> cfblk8/5(cfblk11)
  cfblk9/1(cfblk2) -> cfblk14/1
  cfblk14/1 -> cfblk3/1

== system model_demo/cfblk70 ==
  cfblk1 : Inport
  cfblk13 : Inport  Port=2
  cfblk10 : Abs  SaturateOnIntegerOverflow=off
  cfblk11 : Subsystem
  cfblk12 : Subsystem
  cfblk15 : Delay  SampleTime=1
  cfblk16 : Delay  SampleTime=1
  cfblk3 : DiscreteFilter  SampleTime=1
  cfblk4 : DiscreteIntegrator  ICPrevOutput=DiscIntNeverNeededParam  ICPrevScaledInput=DiscIntNeverNeededParam
  cfblk5 : Delay  DelayLengthSource=Input port  SampleTime=1
      settings: InputPortMap=u0,p1
  cfblk6 : Assignment  DiagnosticForDimensions=Warning  IndexOptions=Index vector (dialog)  Indices=1  OutputSizes=1
  cfblk7 : Squeeze
  cfblk8 : Sin  TimeSource=Use external signal  SampleTime=0
  cfblk9 : Sqrt  Operator=rSqrt  AlgorithmType=Newton-Raphson
  cfblk2 : Outport
  cfblk14 : Outport  Port=2
  wires:
  cfblk6/1 -> cfblk3/1
  cfblk4/1 -> cfblk5/1, cfblk15/1
  cfblk9/1 -> cfblk14/1, cfblk16/1
  cfblk1/1 -> cfblk8/1
  cfblk5/1 -> cfblk9/1
  cfblk3/1 -> cfblk7/1, cfblk5/2
  cfblk13/1 -> cfblk11/1(cfblk1)
  cfblk8/1 -> cfblk10/1, cfblk6/2
  cfblk7/1 -> cfblk2/1, cfblk11/2(cfblk11)
  cfblk11/1(cfblk2) -> cfblk12/2(cfblk7)
  cfblk11/2(cfblk13) -> cfblk12/3(cfblk8)
  cfblk12/1(cfblk2) -> cfblk4/1
  cfblk10/1 -> cfblk6/1
  cfblk15/1 -> cfblk12/1(cfblk1)
  cfblk16/1 -> cfblk11/3(cfblk12)

== system model_demo/cfblk71 ==
  cfblk1 : Inport
  cfblk8 : Inport  Port=2
  cfblk9 : Inport  Port=3
  cfblk3 : DiscreteIntegrator  ICPrevOutput=DiscIntNeverNeededParam  ICPrevScaledInput=DiscIntNeverNeededParam
  cfblk4 : simulink/Discrete/Transfer Fcn Lead or Lag  PoleZ=0.95  ZeroZ=0.75  ICPrevOutput=0.0  ICPrevInput=0.0  DoSatur=off
  cfblk5 : Assignment  DiagnosticForDimensions=Warning  IndexOptions=Index vector (dialog)  Indices=1  OutputSizes=1
  cfblk6 : ComplexToRealImag
  cfblk7 : Constant  Value=[301970440.900590]  SampleTime=1
  cfblk2 : Outport
  wires:
  cfblk9/1 -> cfblk6/1
  cfblk4/1 -> cfblk2/1
  cfblk1/1 -> cfblk5/1
  cfblk7/1 -> cfblk3/1
  cfblk3/1 -> cfblk4/1
  cfblk8/1 -> cfblk5/2

== system model_demo/cfblk72 ==
  cfblk1 : Inport
  cfblk10 : Delay  SampleTime=1
  cfblk11 : Delay  SampleTime=1
  cfblk3 : simulink/Discrete/Transfer Fcn First Order  PoleZ=0.95  ICPrevOutput=0.0  DoSatur=off
  cfblk4 : PropagationDelay  SampleTime=1
  cfblk5 : Sum  Inputs=+-
  cfblk6 : Subsystem
  cfblk7 : Subsystem
  cfblk2 : Outport
  cfblk8 : Outport  Port=2
  cfblk9 : Outport  Port=3
  wires:
  cfblk4/1 -> cfblk6/1(cfblk1), cfblk3/1
  cfblk3/1 -> cfblk2/1
  cfblk1/1 -> cfblk4/1, cfblk6/2(cfblk9), cfblk7/3(cfblk6)
  cfblk7/1(cfblk2) -> cfblk9/1, cfblk10/1
  cfblk6/1(cfblk2) -> cfblk8/1
  cfblk6/2(cfblk11) -> cfblk5/1
  cfblk6/3(cfblk12) -> cfblk5/2
  cfblk5/1 -> cfblk7/1(cfblk1), cfblk7/2(cfblk5), cfblk7/4(cfblk7), cfblk11/1
  cfblk10/1 -> cfblk6/3(cfblk10)
  cfblk11/1 -> cfblk4/2

== system model_demo/cfblk73 ==
  cfblk1 : Inport
  cfblk7 : Inport  Port=2
  cfblk8 : Inport  Port=3
  cfblk10 : Delay  SampleTime=1
  cfblk3 : Sum  Inputs=-+
  cfblk4 : Rounding
  cfblk5 : Sqrt  Operator=rSqrt  AlgorithmType=Newton-Raphson
  cfblk6 : Subsystem
  cfblk9 : Delay  SampleTime=1
  cfblk2 : Outport
  wires:
  cfblk1/1 -> cfblk6/1(cfblk1)
  cfblk4/1 -> cfblk2/1
  cfblk6/1(cfblk2) -> cfblk3/1
  cfblk8/1 -> cfblk6/2(cfblk9)
  cfblk6/2(cfblk12) -> cfblk5/1
  cfblk7/1 -> cfblk3/2
  cfblk5/1 -> cfblk4/1
  cfblk3/1 -> cfblk9/1, cfblk10/1
  cfblk9/1 -> cfblk6/3(cfblk10)
  cfblk10/1 -> cfblk6/4(cfblk11)

== system model_demo/cfblk74 ==
  cfblk1 : Inport
  cfblk3 : simulink/Discrete/Transfer Fcn First Order  PoleZ=0.95  ICPrevOutput=0.0  DoSatur=off
  cfblk4 : DotProduct  OutDataTypeStr=Inherit: Inherit via internal rule
  cfblk5 : Sqrt  Operator=rSqrt  AlgorithmType=Newton-Raphson
  cfblk6 : Abs  SaturateOnIntegerOverflow=off
  cfblk7 : Constant  Value=[-77553052.181357]  SampleTime=1
  cfblk8 : Delay  SampleTime=1
  cfblk2 : Outport
  wires:
  cfblk3/1 -> cfblk2/1
  cfblk4/1 -> cfblk5/1
  cfblk7/1 -> cfblk6/1
  cfblk1/1 -> cfblk4/2
  cfblk6/1 -> cfblk3/1
  cfblk5/1 -> cfblk8/1
  cfblk8/1 -> cfblk4/1

== system model_demo/cfblk75 ==
  cfblk1 : Inport
  cfblk10 : Subsystem
  cfblk11 : Subsystem
  cfblk12 : Subsystem
  cfblk13 : Subsystem
  cfblk14 : Delay  SampleTime=1
  cfblk15 : Delay  SampleTime=1
  cfblk16 : Delay  SampleTime=1
  cfblk3 : DiscreteZeroPole  Poles=[0 0.5]  Gain=1
  cfblk4 : DiscreteIntegrator  ICPrevOutput=DiscIntNeverNeededParam  ICPrevScaledInput=DiscIntNeverNeededParam
  cfblk5 : Sin  TimeSource=Use external signal  SampleTime=0
  cfblk6 : Sqrt
  cfblk7 : Rounding
  cfblk8 : Constant  Value=[572211088.376070]  SampleTime=1
  cfblk9 : Constant  Value=[-377893183.462709]  SampleTime=1
  cfblk2 : Outport
  wires:
  cfblk3/1 -> cfblk6/1
  cfblk4/1 -> cfblk10/1(cfblk1)
  cfblk1/1 -> cfblk4/1
  cfblk11/1(cfblk2) -> cfblk3/1
  cfblk11/2(cfblk16) -> cfblk12/1(cfblk1)
  cfblk8/1 -> cfblk10/2(cfblk8)
  cfblk13/1(cfblk2) -> cfblk2/1
  cfblk6/1 -> cfblk13/1(cfblk1)
  cfblk9/1 -> cfblk11/2(cfblk12), cfblk10/4(cfblk10), cfblk10/5(cfblk11)
  cfblk10/1(cfblk2) -> cfblk12/2(cfblk8)
  cfblk5/1 -> cfblk7/1, cfblk11/5(cfblk15)
  cfblk10/2(cfblk12) -> cfblk11/3(cfblk13)
  cfblk10/3(cfblk13) -> cfblk11/4(cfblk14)
  cfblk12/1(cfblk2) -> cfblk14/1
  cfblk14/1 -> cfblk10/3(cfblk9)
  cfblk13/2(cfblk7) -> cfblk15/1
  cfblk15/1 -> cfblk11/1(cfblk1)
  cfblk7/1 -> cfblk16/1
  cfblk16/1 -> cfblk5/1

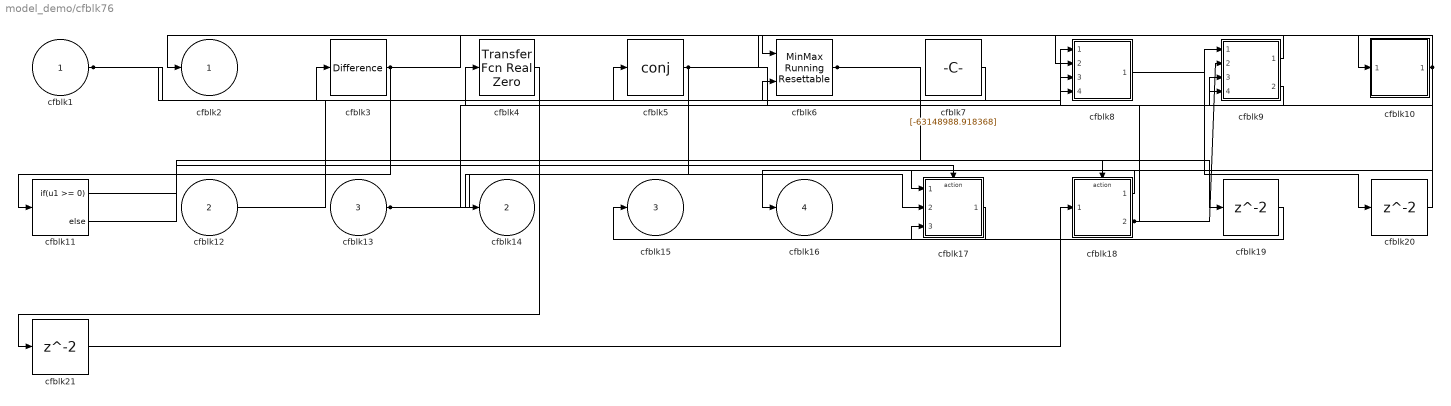
== system model_demo/cfblk76 ==
  cfblk1 : Inport
  cfblk12 : Inport  Port=2
  cfblk13 : Inport  Port=3
  cfblk10 : Subsystem
  cfblk11 : If  IfExpression=u1 >= 0  SampleTime=1
  cfblk17 : Subsystem  TreatAsAtomicUnit=on
  cfblk18 : Subsystem  TreatAsAtomicUnit=on
  cfblk19 : Delay  SampleTime=1
  cfblk20 : Delay  SampleTime=1
  cfblk21 : Delay  SampleTime=1
  cfblk3 : simulink/Discrete/Difference  ICPrevInput=0.0  OutMin=[]  OutMax=[]  OutDataTypeStr=Inherit: Inherit via back propagation  OutDataType=fixdt(1, 16)  OutScaling=2^-10  DoSatur=off
  cfblk4 : simulink/Discrete/Transfer Fcn Real Zero  ZeroZ=0.75  ICPrevInput=0.0  DoSatur=off
  cfblk5 : Math  Operator=conj
  cfblk6 : simulink/Math Operations/MinMax Running Resettable  Function=min  vinit=0.0
  cfblk7 : Constant  Value=[-63148988.918368]  SampleTime=1
  cfblk8 : Subsystem
  cfblk9 : Subsystem
  cfblk2 : Outport
  cfblk14 : Outport  Port=2
  cfblk15 : Outport  Port=3
  cfblk16 : Outport  Port=4
  wires:
  cfblk17/1(cfblk2) -> cfblk15/1
  cfblk18/1(cfblk2) -> cfblk17/1(cfblk1)
  cfblk10/1(cfblk2) -> cfblk2/1, cfblk16/1
  cfblk1/1 -> cfblk3/1, cfblk6/2
  cfblk13/1 -> cfblk17/2(cfblk7), cfblk9/3(cfblk11)
  cfblk3/1 -> cfblk11/1, cfblk8/2(cfblk15)
  cfblk18/2(cfblk8) -> cfblk9/2(cfblk10), cfblk8/4(cfblk17)
  cfblk7/1 -> cfblk5/1
  cfblk12/1 -> cfblk8/1(cfblk1)
  cfblk5/1 -> cfblk14/1, cfblk10/1(cfblk1), cfblk9/4(cfblk12)
  cfblk9/1(cfblk2) -> cfblk6/1
  cfblk6/1 -> cfblk8/3(cfblk16), cfblk19/1
  cfblk9/2(cfblk13) -> cfblk4/1
  cfblk11/1 -> cfblk17/Action
  cfblk11/2 -> cfblk18/Action
  cfblk19/1 -> cfblk17/3(cfblk8)
  cfblk8/1(cfblk2) -> cfblk20/1
  cfblk20/1 -> cfblk9/1(cfblk1)
  cfblk4/1 -> cfblk21/1
  cfblk21/1 -> cfblk18/1(cfblk1)

== system model_demo/cfblk77 ==
  cfblk1 : Inport
  cfblk12 : Inport  Port=2
  cfblk10 : Subsystem
  cfblk11 : If  IfExpression=u1 >= 0  SampleTime=1
  cfblk13 : Subsystem  TreatAsAtomicUnit=on
  cfblk14 : Subsystem  TreatAsAtomicUnit=on
  cfblk15 : Delay  SampleTime=1
  cfblk16 : Delay  SampleTime=1
  cfblk3 : PropagationDelay  SampleTime=1
  cfblk4 : Squeeze
  cfblk5 : Product  Inputs=*
  cfblk6 : Polyval  Coefs=[ +2.081618890e-019, -1.441693666e-014, +4.719686976e-010, -8.536869453e-006, +1.621573104e-001, -8.087801117e+001 ]
  cfblk7 : Constant  Value=[-749646103.857470]  SampleTime=1
  cfblk8 : Subsystem
  cfblk9 : Subsystem
  cfblk2 : Outport
  wires:
  cfblk14/1(cfblk2) -> cfblk13/2(cfblk6), cfblk16/1
  cfblk4/1 -> cfblk9/1(cfblk1)
  cfblk3/1 -> cfblk2/1
  cfblk7/1 -> cfblk4/1, cfblk14/4(cfblk17), cfblk13/3(cfblk7)
  cfblk9/1(cfblk2) -> cfblk10/2(cfblk8)
  cfblk10/1(cfblk2) -> cfblk14/1(cfblk1)
  cfblk6/1 -> cfblk3/1
  cfblk1/1 -> cfblk3/2
  cfblk8/1(cfblk2) -> cfblk5/1
  cfblk12/1 -> cfblk8/1(cfblk1)
  cfblk13/1(cfblk2) -> cfblk8/2(cfblk14), cfblk8/4(cfblk16)
  cfblk9/2(cfblk11) -> cfblk6/1
  cfblk9/3(cfblk12) -> cfblk14/2(cfblk15)
  cfblk9/4(cfblk13) -> cfblk8/3(cfblk15)
  cfblk9/5(cfblk14) -> cfblk14/3(cfblk16), cfblk13/1(cfblk1)
  cfblk11/1 -> cfblk13/Action
  cfblk11/2 -> cfblk14/Action
  cfblk5/1 -> cfblk15/1
  cfblk15/1 -> cfblk10/1(cfblk1)
  cfblk16/1 -> cfblk11/1

== system model_demo/cfblk78 ==
  cfblk1 : Inport
  cfblk9 : Inport  Port=2
  cfblk10 : Inport  Port=3
  cfblk11 : Inport  Port=4
  cfblk12 : Inport  Port=5
  cfblk13 : Inport  Port=6
  cfblk14 : Inport  Port=7
  cfblk3 : simulink/Discrete/Tapped Delay  vinit=0.0  samptime=-1  NumDelays=1  DelayOrder=Oldest  includeCurrent=off
  cfblk4 : simulink/Discrete/Transfer Fcn Real Zero  ZeroZ=0.75  ICPrevInput=0.0  DoSatur=off
  cfblk5 : Gain  Gain=[174515567.740750]
  cfblk6 : Constant  Value=[-431350872.321189]  SampleTime=1
  cfblk7 : Subsystem
  cfblk8 : Subsystem
  cfblk2 : Outport
  wires:
  cfblk10/1 -> cfblk2/1
  cfblk1/1 -> cfblk8/1(cfblk1)
  cfblk5/1 -> cfblk7/1(cfblk1)
  cfblk11/1 -> cfblk4/1
  cfblk4/1 -> cfblk8/2(cfblk14)
  cfblk12/1 -> cfblk3/1
  cfblk9/1 -> cfblk7/2(cfblk10)
  cfblk14/1 -> cfblk5/1

== system model_demo/cfblk79 ==
  cfblk1 : Inport
  cfblk13 : Inport  Port=2
  cfblk10 : Constant  Value=[-37990502.760676]  SampleTime=1
  cfblk11 : Constant  Value=[-533394616.075941]  SampleTime=1
  cfblk12 : Subsystem
  cfblk14 : Delay  SampleTime=1
  cfblk3 : DiscreteZeroPole  Poles=[0 0.5]  Gain=1
  cfblk4 : simulink/Discrete/Difference  ICPrevInput=0.0  OutMin=[]  OutMax=[]  OutDataTypeStr=Inherit: Inherit via back propagation  OutDataType=fixdt(1, 16)  OutScaling=2^-10  DoSatur=off
  cfblk5 : DiscreteStateSpace
  cfblk6 : simulink/Discrete/Tapped Delay  vinit=0.0  samptime=-1  NumDelays=1  DelayOrder=Oldest  includeCurrent=off
  cfblk7 : ComplexToMagnitudeAngle
  cfblk8 : Sum  Inputs=+-
  cfblk9 : simulink/Math Operations/MinMax Running Resettable  Function=min  vinit=0.0
  cfblk2 : Outport
  wires:
  cfblk13/1 -> cfblk3/1
  cfblk3/1 -> cfblk2/1
  cfblk9/1 -> cfblk5/1
  cfblk1/1 -> cfblk12/1(cfblk1)
  cfblk10/1 -> cfblk4/1
  cfblk11/1 -> cfblk8/1
  cfblk4/1 -> cfblk6/1
  cfblk8/1 -> cfblk7/1
  cfblk7/1 -> cfblk9/2
  cfblk12/1(cfblk2) -> cfblk8/2
  cfblk5/1 -> cfblk14/1
  cfblk14/1 -> cfblk9/1

== system model_demo/cfblk80 ==
  cfblk1 : Inport
  cfblk10 : Inport  Port=2
  cfblk12 : Delay  SampleTime=1
  cfblk13 : Delay  SampleTime=1
  cfblk14 : Delay  SampleTime=1
  cfblk3 : DiscreteTransferFcn  SampleTime=1
  cfblk4 : Rounding
  cfblk5 : Sqrt
  cfblk6 : Subsystem
  cfblk7 : Subsystem
  cfblk8 : Subsystem
  cfblk9 : Subsystem
  cfblk2 : Outport
  cfblk11 : Outport  Port=2
  wires:
  cfblk10/1 -> cfblk9/1(cfblk1)
  cfblk5/1 -> cfblk9/2(cfblk12), cfblk8/3(cfblk10)
  cfblk6/1(cfblk2) -> cfblk3/1
  cfblk7/1(cfblk2) -> cfblk4/1, cfblk5/1
  cfblk6/2(cfblk11) -> cfblk11/1
  cfblk9/1(cfblk2) -> cfblk8/2(cfblk9)
  cfblk1/1 -> cfblk7/2(cfblk9)
  cfblk8/1(cfblk2) -> cfblk6/1(cfblk1)
  cfblk8/3(cfblk12) -> cfblk2/1
  cfblk4/1 -> cfblk12/1
  cfblk12/1 -> cfblk7/1(cfblk1)
  cfblk3/1 -> cfblk13/1
  cfblk13/1 -> cfblk8/1(cfblk1)
  cfblk8/2(cfblk11) -> cfblk14/1
  cfblk14/1 -> cfblk9/3(cfblk13)

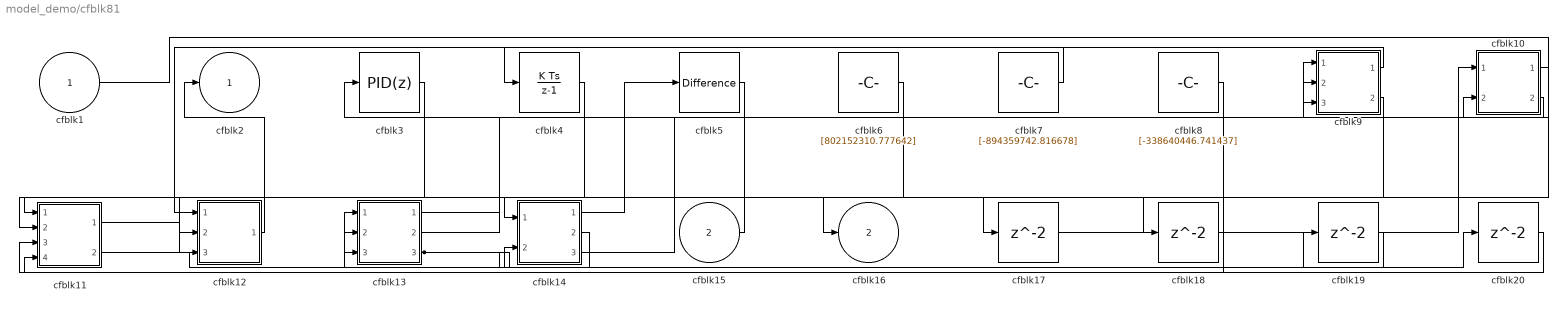
== system model_demo/cfblk81 ==
  cfblk1 : Inport
  cfblk15 : Inport  Port=2
  cfblk10 : Subsystem
  cfblk11 : Subsystem
  cfblk12 : Subsystem
  cfblk13 : Subsystem
  cfblk14 : Subsystem
  cfblk{17..20} (4 alike) : Delay  SampleTime=1
  cfblk3 : slpidlib/PID Controller  Controller=PID  Form=Parallel  TimeDomain=Discrete-time  UseExternalTs=off  SampleTime=1  IntegratorMethod=Forward Euler  FilterMethod=Forward Euler  ControllerParametersSource=internal  P=1  I=1  UseKiTs=off  D=0  N=100  UseFilter=on  TunerSelectOption=Transfer Function Based (PID Tuner App)  InitialConditionSource=internal  InitialConditionForIntegrator=0  InitialConditionForFilter=0  DifferentiatorICPrevScaledInput=0  ExternalReset=none  TrackingMode=off  Kt=1  LimitOutput=off  SatLimitsSource=internal  UpperSaturationLimit=inf  LowerSaturationLimit=-inf  LinearizeAsGain=off  AntiWindupMode=none  Kb=1  LimitIntegrator=off  UpperIntegratorSaturationLimit=inf  LowerIntegratorSaturationLimit=-inf  POutMin=[]  POutMax=[]  IOutMin=[]  IOutMax=[]  DOutMin=[]  DOutMax=[]  NOutMin=[]  NOutMax=[]  SumOutMin=[]  SumOutMax=[]  SaturationOutMin=[]  SaturationOutMax=[]  PParamMin=[]  PParamMax=[]  IParamMin=[]  IParamMax=[]  DParamMin=[]  DParamMax=[]  NParamMin=[]  NParamMax=[]  KbParamMin=[]  KbParamMax=[]  KtParamMin=[]  KtParamMax=[]  KbOutMin=[]  KbOutMax=[]  KtOutMin=[]  KtOutMax=[]  IntegratorOutMin=[]  IntegratorOutMax=[]  FilterOutMin=[]  FilterOutMax=[]  SumI1OutMin=[]  SumI1OutMax=[]  SumI2OutMin=[]  SumI2OutMax=[]  SumI3OutMin=[]  SumI3OutMax=[]  SumI4OutMin=[]  SumI4OutMax=[]  SumDOutMin=[]  SumDOutMax=[]  DifferentiatorOutMin=[]  DifferentiatorOutMax=[]  FilterDiffOutCoefMin=[]  FilterDiffOutCoefMax=[]  ReciprocalOutMin=[]  ReciprocalOutMax=[]  SumDenOutMin=[]  SumDenOutMax=[]  SumNumOutMin=[]  SumNumOutMax=[]  DivideOutMin=[]  DivideOutMax=[]  UdiffTsProdOutMin=[]  UdiffTsProdOutMax=[]  NTsProdOutMin=[]  NTsProdOutMax=[]  UintegralTsProdOutMin=[]  UintegralTsProdOutMax=[]  UngainTsProdOutMin=[]  UngainTsProdOutMax=[]  ClampingZeroOutDataTypeStr=Inherit: Inherit via back propagation  ClampingZeroOutMin=[]  ClampingZeroOutMax=[]  FilterDenConstantOutDataTypeStr=Inherit: Inherit via back propagation  FilterDenConstantOutMin=[]  FilterDenConstantOutMax=[]  PCopyOutDataTypeStr=Inherit: Inherit via back propagation  PCopyOutMin=[]  PCopyOutMax=[]  NCopyOutDataTypeStr=Inherit: Inherit via back propagation  NCopyOutMin=[]  NCopyOutMax=[]  IntegratorContinuousStateAttributes=''  IntegratorStateMustResolveToSignalObject=off  IntegratorRTWStateStorageClass=Auto  FilterContinuousStateAttributes=''  FilterStateMustResolveToSignalObject=off  FilterRTWStateStorageClass=Auto  ParallelPVariant=InternalParameters  IdealPVariant=Disabled  IVariant=InternalParameters  DVariant=InternalParameters  IntegratorVariant=Discrete  SatVariant=Disabled  AWVariant=Passthrough  PCopyVariant=Disabled  TRVariant=Disabled  FdbkBlocksVariant=Forward  IdealPFdbkVariant=Disabled  SatFdbkVariant=Disabled  DerivativeFilterVariant=ForwardEulerFilter  NVariant=InternalParameters  NCopyVariant=Disabled  FilterICVariant=InternalICsFilter  IntegratorICVariant=InternalICs  ExternalResetVariant=Disabled  TRSumVariant=Passthrough  SumFdbkVariant=Disabled  SumVariant=Sum_PID  TsampFilterVariant=InternalTs  TsampNgainVariant=Passthrough  TsampIntegralVariant=Disabled_SignalSpec  ExternalSaturationOutDataTypeStr=Inherit: Same as second input
      settings: LibrarySourceBlock=simulink/Discrete/Discrete PID Controller
  cfblk4 : DiscreteIntegrator  ICPrevOutput=DiscIntNeverNeededParam  ICPrevScaledInput=DiscIntNeverNeededParam
  cfblk5 : simulink/Discrete/Difference  ICPrevInput=0.0  OutMin=[]  OutMax=[]  OutDataTypeStr=Inherit: Inherit via back propagation  OutDataType=fixdt(1, 16)  OutScaling=2^-10  DoSatur=off
  cfblk6 : Constant  Value=[802152310.777642]  SampleTime=1
  cfblk7 : Constant  Value=[-894359742.816678]  SampleTime=1
  cfblk8 : Constant  Value=[-338640446.741437]  SampleTime=1
  cfblk9 : Subsystem
  cfblk2 : Outport
  cfblk16 : Outport  Port=2
  wires:
  cfblk12/1(cfblk2) -> cfblk2/1
  cfblk9/1(cfblk2) -> cfblk12/1(cfblk1)
  cfblk4/1 -> cfblk14/1(cfblk1)
  cfblk8/1 -> cfblk13/1(cfblk1)
  cfblk14/1(cfblk2) -> cfblk5/1
  cfblk5/1 -> cfblk11/1(cfblk1)
  cfblk7/1 -> cfblk4/1
  cfblk11/1(cfblk2) -> cfblk16/1
  cfblk15/1 -> cfblk3/1
  cfblk1/1 -> cfblk10/2(cfblk6)
  cfblk11/2(cfblk11) -> cfblk13/2(cfblk10)
  cfblk6/1 -> cfblk11/2(cfblk8)
  cfblk10/1(cfblk2) -> cfblk12/2(cfblk16)
  cfblk14/2(cfblk15) -> cfblk13/3(cfblk11)
  cfblk13/1(cfblk2) -> cfblk9/1(cfblk1)
  cfblk14/3(cfblk16) -> cfblk9/2(cfblk7)
  cfblk10/2(cfblk7) -> cfblk9/3(cfblk8)
  cfblk13/3(cfblk13) -> cfblk19/1, cfblk20/1
  cfblk3/1 -> cfblk12/3(cfblk17)
  cfblk9/2(cfblk9) -> cfblk17/1
  cfblk17/1 -> cfblk10/1(cfblk1)
  cfblk13/2(cfblk12) -> cfblk18/1
  cfblk18/1 -> cfblk11/3(cfblk9)
  cfblk19/1 -> cfblk14/2(cfblk14)
  cfblk20/1 -> cfblk11/4(cfblk10)
